simulink model "WGS_84"  (R2024b)
settings: Solver=VariableStepAuto  StartTime=0.0  StopTime=10.0  RelTol=1e-3
settings Model: Creator=satvik_sh  LastModifiedBy=satvik_sh

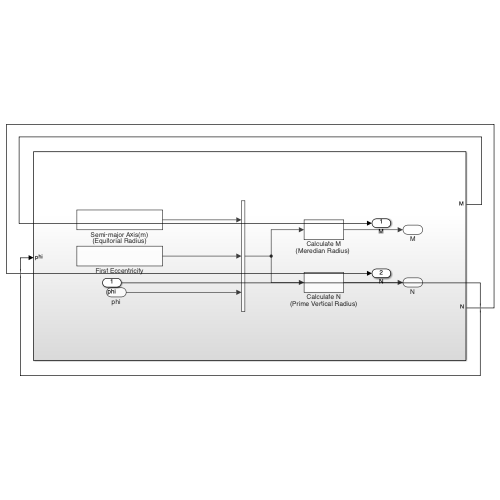
[thumbnail: Simulink's stored preview of the top-level diagram]
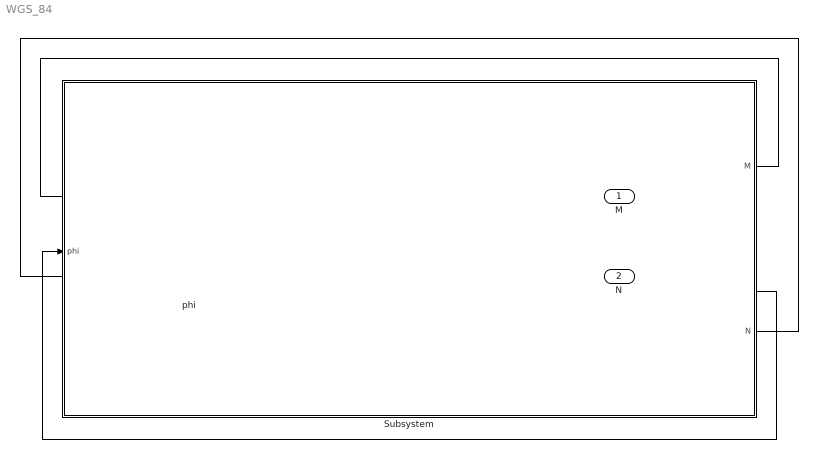
== system WGS_84 ==
  phi : Inport
  Subsystem : Subsystem
  M : Outport
  N : Outport  Port=2
  wires:
  phi/1 -> Subsystem/1(phi)
  Subsystem/1(M) -> M/1
  Subsystem/2(N) -> N/1

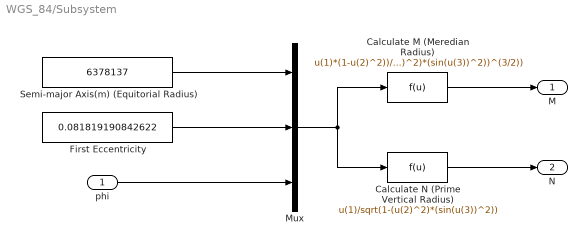
== system WGS_84/Subsystem ==
  phi : Inport
  "Calculate M (Meredian Radius) " : Fcn  Expr=u(1)*(1-u(2)^2))/((1-u(2)^2)*(sin(u(3))^2))^(3/2))
  Calculate N (Prime Vertical Radius) : Fcn  Expr=u(1)/sqrt(1-(u(2)^2)*(sin(u(3))^2))
  First Eccentricity : Constant  Value=0.081819190842622
  Mux : Mux  Inputs=3
  Semi-major Axis(m) (Equitorial Radius) : Constant  Value=6378137
  M : Outport
  N : Outport  Port=2
  wires:
  First Eccentricity/1 -> Mux/2
  phi/1 -> Mux/3
  Calculate N (Prime Vertical Radius)/1 -> N/1
  Mux/1 -> Calculate N (Prime Vertical Radius)/1, "Calculate M (Meredian Radius) "/1
  "Calculate M (Meredian Radius) "/1 -> M/1
  Semi-major Axis(m) (Equitorial Radius)/1 -> Mux/1
